simulink model "MAS_C4_Example3"  (R2021b)
settings: Solver=VariableStepAuto  StartTime=0.0  StopTime=1000  RelTol=1e-3
libraries: cstblocks x6
settings Model: Creator=lenovo  LastModifiedBy=lenovo

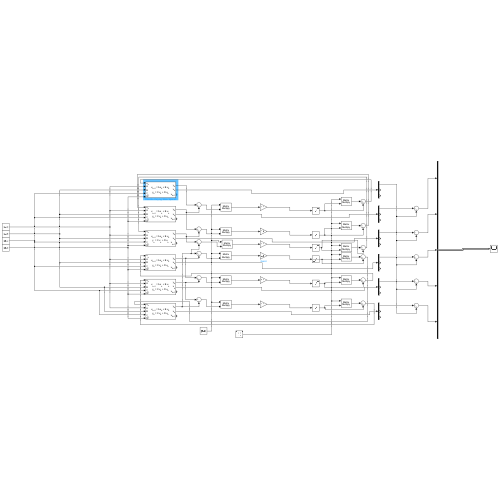
[thumbnail: Simulink's stored preview of the top-level diagram]
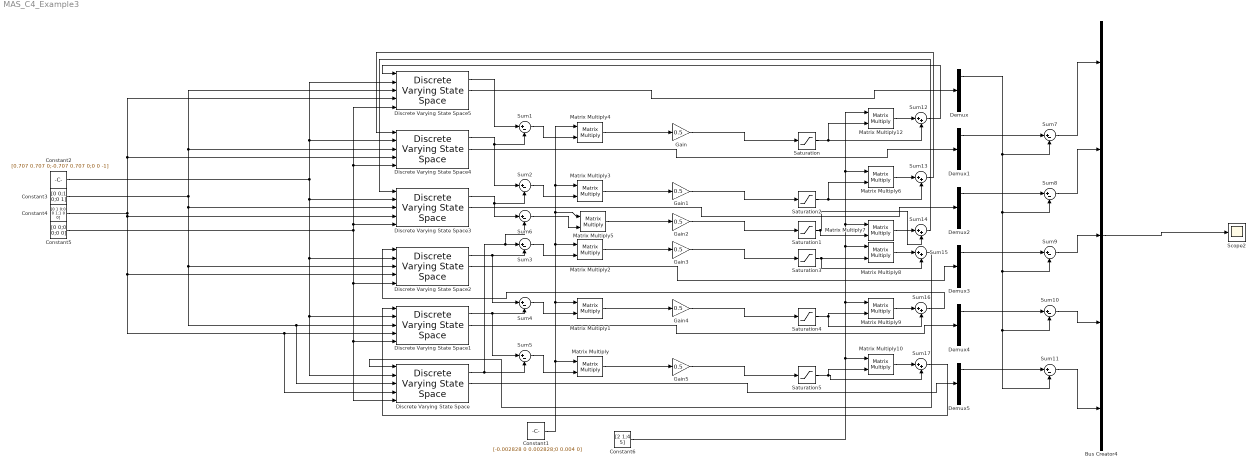
== system MAS_C4_Example3 ==
  Bus Creator4 : BusCreator  Inputs=5
  Constant1 : Constant  Value=[-0.002828 0 0.002828;0 0.004 0]  VectorParams1D=off
  Constant2 : Constant  Value=[0.707 0.707 0;-0.707 0.707 0;0 0 -1]
  Constant3 : Constant  Value=[0 0;1 0;0 1]
  Constant4 : Constant  Value=[0 1 0;0 0 1;1 0 0]  VectorParams1D=off
  Constant5 : Constant  Value=[0 0;0 0;0 0]  VectorParams1D=off
  Constant6 : Constant  Value=[2 1;4 5]  VectorParams1D=off
  Demux{,1..5} (6 alike) : Demux  Outputs=3
  Discrete Varying State Space{,1..5} (6 alike) : cstblocks/Linear Parameter Varying/Discrete Varying State Space  x0=0  Ts=-1  OutputX=on  OutputDX=on
      settings: SourceProductBaseCode=CT
  Gain{,1..5} (6 alike) : Gain  Gain=0.5
  Matrix Multiply{,1..10,12} (12 alike) : Product  Multiplication=Matrix(*)
  Saturation{,1..5} (6 alike) : Saturate  UpperLimit=1  LowerLimit=-1
  Scope2 : Scope
  Sum{1..11} (11 alike) : Sum  Inputs=|+-
  Sum{12..17} (6 alike) : Sum  Inputs=|++
  wires:
  Bus Creator4/1 -> Scope2/1
  Constant2/1 -> Discrete Varying State Space3/2, Discrete Varying State Space2/2, Discrete Varying State Space1/2, Discrete Varying State Space/2, Discrete Varying State Space5/2, Discrete Varying State Space4/2
  Constant3/1 -> Discrete Varying State Space3/3, Discrete Varying State Space2/3, Discrete Varying State Space1/3, Discrete Varying State Space/3, Discrete Varying State Space5/3, Discrete Varying State Space4/3
  Constant4/1 -> Discrete Varying State Space3/4, Discrete Varying State Space2/4, Discrete Varying State Space1/4, Discrete Varying State Space/4, Discrete Varying State Space5/4, Discrete Varying State Space4/4
  Constant5/1 -> Discrete Varying State Space2/5, Discrete Varying State Space1/5, Discrete Varying State Space/5, Discrete Varying State Space3/5, Discrete Varying State Space5/5, Discrete Varying State Space4/5
  Discrete Varying State Space2/2 -> Demux3/1
  Discrete Varying State Space1/2 -> Demux4/1
  Discrete Varying State Space/2 -> Demux5/1
  Discrete Varying State Space3/2 -> Demux2/1
  Discrete Varying State Space4/2 -> Demux1/1
  Discrete Varying State Space5/2 -> Demux/1
  Saturation4/1 -> Matrix Multiply9/2, Sum16/2
  Saturation3/1 -> Matrix Multiply8/2, Sum15/2
  Saturation2/1 -> Sum13/2, Matrix Multiply6/2
  Constant1/1 -> Matrix Multiply5/1, Matrix Multiply4/1, Matrix Multiply3/1, Matrix Multiply2/1, Matrix Multiply1/1, Matrix Multiply/1
  Saturation5/1 -> Sum17/2, Matrix Multiply10/2
  Discrete Varying State Space1/1 -> Sum5/1, Sum4/2
  Discrete Varying State Space/1 -> Sum3/1, Sum6/2, Sum5/2
  Discrete Varying State Space2/1 -> Sum4/1, Sum3/2
  Discrete Varying State Space3/1 -> Sum6/1, Sum2/2
  Discrete Varying State Space4/1 -> Sum2/1, Sum1/2
  Discrete Varying State Space5/1 -> Sum1/1
  Sum1/1 -> Matrix Multiply4/2
  Sum2/1 -> Matrix Multiply3/2
  Sum3/1 -> Matrix Multiply2/2
  Sum4/1 -> Matrix Multiply1/2
  Sum5/1 -> Matrix Multiply/2
  Demux3/1 -> Sum9/1
  Demux4/1 -> Sum10/1
  Demux5/1 -> Sum11/1
  Demux2/1 -> Sum8/1
  Demux1/1 -> Sum7/1
  Demux/1 -> Sum8/2, Sum11/2, Sum10/2, Sum9/2, Sum7/2
  Sum9/1 -> Bus Creator4/3
  Sum8/1 -> Bus Creator4/2
  Sum7/1 -> Bus Creator4/1
  Sum11/1 -> Bus Creator4/5
  Sum10/1 -> Bus Creator4/4
  Sum6/1 -> Matrix Multiply5/2
  Saturation1/1 -> Matrix Multiply7/2, Sum14/2
  Constant6/1 -> Matrix Multiply10/1, Matrix Multiply9/1, Matrix Multiply8/1, Matrix Multiply7/1, Matrix Multiply6/1, Matrix Multiply12/1
  Saturation/1 -> Sum12/2, Matrix Multiply12/2
  Matrix Multiply12/1 -> Sum12/1
  Sum12/1 -> Discrete Varying State Space5/1
  Matrix Multiply9/1 -> Sum16/1
  Matrix Multiply10/1 -> Sum17/1
  Matrix Multiply8/1 -> Sum15/1
  Matrix Multiply7/1 -> Sum14/1
  Matrix Multiply6/1 -> Sum13/1
  Sum13/1 -> Discrete Varying State Space4/1
  Sum14/1 -> Discrete Varying State Space3/1
  Sum15/1 -> Discrete Varying State Space/1
  Sum16/1 -> Discrete Varying State Space2/1
  Sum17/1 -> Discrete Varying State Space1/1
  Matrix Multiply/1 -> Gain5/1
  Matrix Multiply1/1 -> Gain4/1
  Matrix Multiply2/1 -> Gain3/1
  Matrix Multiply5/1 -> Gain2/1
  Matrix Multiply3/1 -> Gain1/1
  Matrix Multiply4/1 -> Gain/1
  Gain/1 -> Saturation/1
  Gain1/1 -> Saturation2/1
  Gain2/1 -> Saturation1/1
  Gain3/1 -> Saturation3/1
  Gain4/1 -> Saturation4/1
  Gain5/1 -> Saturation5/1
